simulink model "ResonantConverter_GaN"  (R2016a)
settings: Solver=VariableStepAuto  StartTime=0.0  StopTime=0.1  FixedStep=1e-6  RelTol=1e-3
libraries: powerlib x142, dspstat3 x22, powerlib_meascontrol x13
(part 1 of 2)
settings Model: Creator=syf  LastModifiedBy=syf
settings SolverCC: AutoInsertRateTranBlk=on

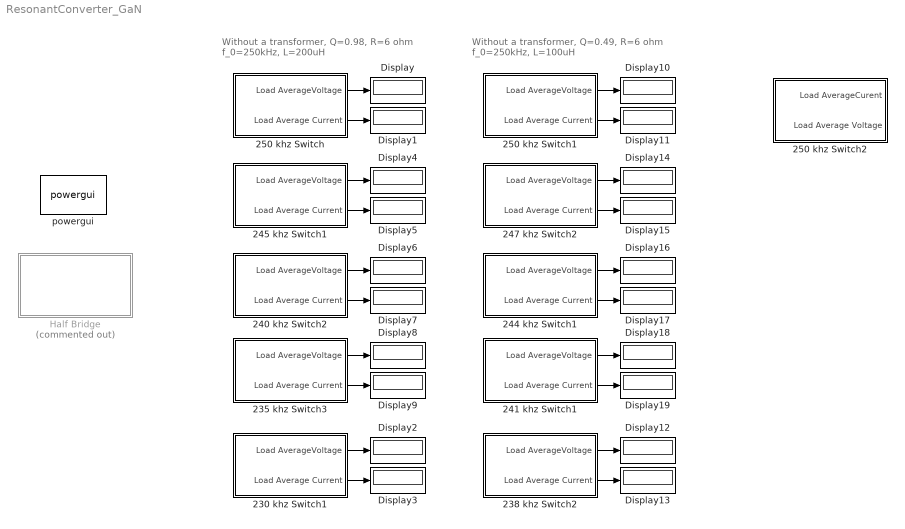
== system ResonantConverter_GaN ==
  note: Without a transformer, Q=0.98, R=6 ohm
      | f_0=250kHz, L=200uH
  note: Without a transformer, Q=0.49, R=6 ohm
      | f_0=250kHz, L=100uH
  230 khz Switch1 : Subsystem
  235 khz Switch3 : Subsystem
  238 khz Switch2 : Subsystem
  240 khz Switch2 : Subsystem
  241 khz Switch1 : Subsystem
  244 khz Switch1 : Subsystem
  245 khz Switch1 : Subsystem
  247 khz Switch2 : Subsystem
  250 khz Switch : Subsystem
  250 khz Switch1 : Subsystem
  250 khz Switch2 : Subsystem
  Display{,1..19} (20 alike) : Display
  Half Bridge : Subsystem  Commented=on
  powergui : powerlib/powergui  Priority=1  SimulationMode=Continuous  SolverType=Tustin/Backward Euler (TBE)  SampleTime=50e-6  frequency=60  SPID=on  DisableSnubberDevices=on  DisableRonSwitches=off  DisableVfSwitches=off  SwTol=0  DisplayEquations=off  Interpol=off  ExternalGateDelay=off  methode=off  Ts=10  FunctionMessages=off  echomessages=off  HookPort=off  EnableUseOfTLC=off  x0status=blocks  frequencyindice=0  Pbase=100e6  ErrMax=1e-4  Iterations=50  UnitsV=kV  UnitsW=MW  buscounter=0  RestoreLinks=warning  ResistiveCurrentMeasurement=off  Frange=[0:2:500]  Ylog=off  Xlog=on  ShowGrid=off  save=off  variable=ZData  structure=0  ZoomFFT=off  StartTime=0.0  cycles=1  DisplayStyle=1  fundamental=60  FreqAxis=off  MaxFrequency=1000  frequencyindicesteady=1  RmsSteady=1  display=off
  wires:
  250 khz Switch/2(Load Average Current) -> Display1/1
  250 khz Switch/1(Load AverageVoltage) -> Display/1
  230 khz Switch1/2(Load Average Current) -> Display3/1
  230 khz Switch1/1(Load AverageVoltage) -> Display2/1
  245 khz Switch1/2(Load Average Current) -> Display5/1
  245 khz Switch1/1(Load AverageVoltage) -> Display4/1
  240 khz Switch2/2(Load Average Current) -> Display7/1
  240 khz Switch2/1(Load AverageVoltage) -> Display6/1
  235 khz Switch3/2(Load Average Current) -> Display9/1
  235 khz Switch3/1(Load AverageVoltage) -> Display8/1
  250 khz Switch1/2(Load Average Current) -> Display11/1
  250 khz Switch1/1(Load AverageVoltage) -> Display10/1
  238 khz Switch2/2(Load Average Current) -> Display13/1
  238 khz Switch2/1(Load AverageVoltage) -> Display12/1
  247 khz Switch2/2(Load Average Current) -> Display15/1
  247 khz Switch2/1(Load AverageVoltage) -> Display14/1
  244 khz Switch1/2(Load Average Current) -> Display17/1
  244 khz Switch1/1(Load AverageVoltage) -> Display16/1
  241 khz Switch1/2(Load Average Current) -> Display19/1
  241 khz Switch1/1(Load AverageVoltage) -> Display18/1

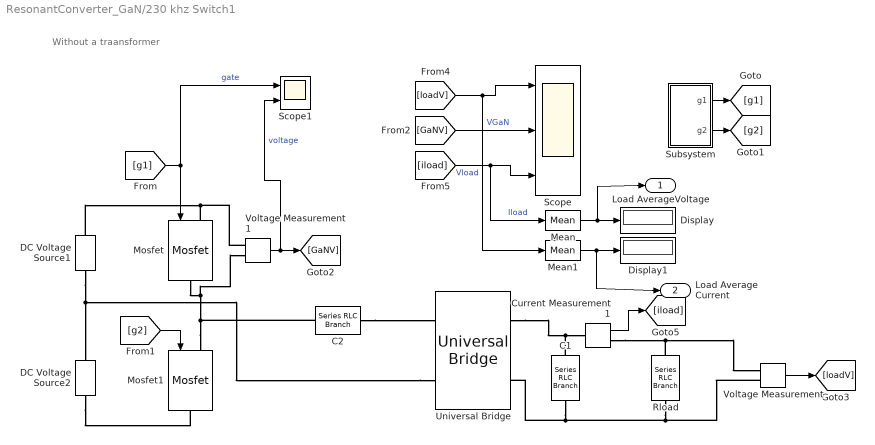
== system ResonantConverter_GaN/230 khz Switch1 ==
  note: Without a traansformer
  C1 : powerlib/Elements/Series RLC Branch  LConnTagsString=__new0  RConnTagsString=__new0  BranchType=C  Resistance=1  Inductance=1e-3  SetiL0=off  InitialCurrent=0  Capacitance=47e-6  Setx0=off  InitialVoltage=0  Measurements=None
  C2 : powerlib/Elements/Series RLC Branch  LConnTagsString=__new0  RConnTagsString=__new0  BranchType=LC  Resistance=1  Inductance=200e-6  SetiL0=off  InitialCurrent=0  Capacitance=0.02027e-7  Setx0=off  InitialVoltage=0  Measurements=None
  Current Measurement1 : powerlib/Measurements/Current Measurement  PhasorSimulation=off  OutputType=Complex  PSBequivalent=0
  DC Voltage Source1 : powerlib/Electrical Sources/DC Voltage Source  Amplitude=190  Measurements=None
  DC Voltage Source2 : powerlib/Electrical Sources/DC Voltage Source  Amplitude=190  Measurements=None
  Display : Display
  Display1 : Display
  Mean : dspstat3/Mean  run=off  reset_popup=None  InputProcessing=Columns as channels (frame based)  directionMode=Each column  dimension=1  roiEnable=off  roiType=Rectangles  roiPortion=Entire ROI  roiOutput=Individual statistics for each ROI  roiFlag=off  outputDataTypeStr=Inherit: Same as accumulator  outputLastDataTypeStr=Inherit: Same as accumulator  outputMin=[]  outputMax=[]  roundingMode=Floor  overflowMode=off
  Mean1 : dspstat3/Mean  run=off  reset_popup=None  InputProcessing=Columns as channels (frame based)  directionMode=Each column  dimension=1  roiEnable=off  roiType=Rectangles  roiPortion=Entire ROI  roiOutput=Individual statistics for each ROI  roiFlag=off  outputDataTypeStr=Inherit: Same as accumulator  outputLastDataTypeStr=Inherit: Same as accumulator  outputMin=[]  outputMax=[]  roundingMode=Floor  overflowMode=off
  Mosfet : powerlib/Power Electronics/Mosfet  Ron=130e-3  Lon=0  Rd=0.25  Vfd=2.2  IC=0  Rs=1e5  Cs=inf  Measurements=off
  Mosfet1 : powerlib/Power Electronics/Mosfet  Ron=130e-3  Lon=0  Rd=0.25  Vfd=2.2  IC=0  Rs=1e5  Cs=inf  Measurements=off
  Rload : powerlib/Elements/Series RLC Branch  LConnTagsString=__new0  RConnTagsString=__new0  BranchType=R  Resistance=6  Inductance=1e-3  SetiL0=off  InitialCurrent=0  Capacitance=1e-6  Setx0=off  InitialVoltage=0  Measurements=None
  Scope : Scope  NumInputPorts=3
  Scope1 : Scope  NumInputPorts=2
  Subsystem : Subsystem
  Universal Bridge : powerlib/Power Electronics/Universal Bridge  Arms=2  SnubberResistance=1e5  SnubberCapacitance=inf  Device=Diodes  Ron=1e-3  Lon=0  ForwardVoltages="[  0  0  ]"  ForwardVoltage=0  GTOparameters=[ 10e-6 , 20e-6 ]  IGBTparameters=[ 1e-6 , 2e-6 ]  Measurements=None  Measurements_2=None  converterType=Rectifier
  Voltage Measurement : powerlib/Measurements/Voltage Measurement  PhasorSimulation=off  OutputType=Complex  PSBequivalent=0
  Voltage Measurement1 : powerlib/Measurements/Voltage Measurement  PhasorSimulation=off  OutputType=Complex  PSBequivalent=0
  Load AverageVoltage : Outport
  Load Average Current : Outport  Port=2
  wires:
  Mean1/1 -> Display1/1, Load Average Current/1
  Current Measurement1/1 -> [iload]
  Voltage Measurement1/1 -> Scope1/2, [GaNV]  "voltage"
  [g2] -> Mosfet1/1
  Voltage Measurement/1 -> [loadV]
  [GaNV] -> Scope/2  "VGaN"
  [loadV] -> Scope/1, Mean1/1  "Vload"
  [iload] -> Scope/3, Mean/1  "Iload"
  [g1] -> Scope1/1, Mosfet/1  "gate"
  Subsystem/2(g2) -> [g2]
  Subsystem/1("g1 ") -> [g1]
  Mean/1 -> Display/1, Load AverageVoltage/1
  connections:
  DC Voltage Source2/LConn1 -- Mosfet1/RConn1
  Current Measurement1/RConn1 -- Voltage Measurement/LConn1 -- Rload/LConn1
  Universal Bridge/LConn2 -- DC Voltage Source1/LConn1 -- DC Voltage Source2/RConn1
  DC Voltage Source1/RConn1 -- Voltage Measurement1/LConn1 -- Mosfet/LConn1
  Mosfet1/LConn1 -- C2/LConn1 -- Voltage Measurement1/LConn2 -- Mosfet/RConn1
  C1/LConn1 -- Universal Bridge/RConn1 -- Current Measurement1/LConn1
  C1/RConn1 -- Universal Bridge/RConn2 -- Voltage Measurement/LConn2 -- Rload/RConn1
  C2/RConn1 -- Universal Bridge/LConn1

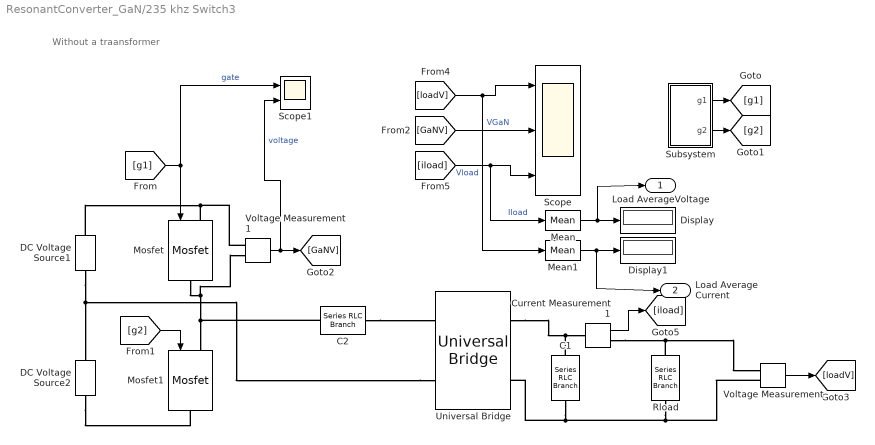
== system ResonantConverter_GaN/235 khz Switch3 ==
  note: Without a traansformer
  C1 : powerlib/Elements/Series RLC Branch  LConnTagsString=__new0  RConnTagsString=__new0  BranchType=C  Resistance=1  Inductance=1e-3  SetiL0=off  InitialCurrent=0  Capacitance=47e-6  Setx0=off  InitialVoltage=0  Measurements=None
  C2 : powerlib/Elements/Series RLC Branch  LConnTagsString=__new0  RConnTagsString=__new0  BranchType=LC  Resistance=1  Inductance=200e-6  SetiL0=off  InitialCurrent=0  Capacitance=0.02027e-7  Setx0=off  InitialVoltage=0  Measurements=None
  Current Measurement1 : powerlib/Measurements/Current Measurement  PhasorSimulation=off  OutputType=Complex  PSBequivalent=0
  DC Voltage Source1 : powerlib/Electrical Sources/DC Voltage Source  Amplitude=190  Measurements=None
  DC Voltage Source2 : powerlib/Electrical Sources/DC Voltage Source  Amplitude=190  Measurements=None
  Display : Display
  Display1 : Display
  Mean : dspstat3/Mean  run=off  reset_popup=None  InputProcessing=Columns as channels (frame based)  directionMode=Each column  dimension=1  roiEnable=off  roiType=Rectangles  roiPortion=Entire ROI  roiOutput=Individual statistics for each ROI  roiFlag=off  outputDataTypeStr=Inherit: Same as accumulator  outputLastDataTypeStr=Inherit: Same as accumulator  outputMin=[]  outputMax=[]  roundingMode=Floor  overflowMode=off
  Mean1 : dspstat3/Mean  run=off  reset_popup=None  InputProcessing=Columns as channels (frame based)  directionMode=Each column  dimension=1  roiEnable=off  roiType=Rectangles  roiPortion=Entire ROI  roiOutput=Individual statistics for each ROI  roiFlag=off  outputDataTypeStr=Inherit: Same as accumulator  outputLastDataTypeStr=Inherit: Same as accumulator  outputMin=[]  outputMax=[]  roundingMode=Floor  overflowMode=off
  Mosfet : powerlib/Power Electronics/Mosfet  Ron=130e-3  Lon=0  Rd=0.25  Vfd=2.2  IC=0  Rs=1e5  Cs=inf  Measurements=off
  Mosfet1 : powerlib/Power Electronics/Mosfet  Ron=130e-3  Lon=0  Rd=0.25  Vfd=2.2  IC=0  Rs=1e5  Cs=inf  Measurements=off
  Rload : powerlib/Elements/Series RLC Branch  LConnTagsString=__new0  RConnTagsString=__new0  BranchType=R  Resistance=6  Inductance=1e-3  SetiL0=off  InitialCurrent=0  Capacitance=1e-6  Setx0=off  InitialVoltage=0  Measurements=None
  Scope : Scope  NumInputPorts=3
  Scope1 : Scope  NumInputPorts=2
  Subsystem : Subsystem
  Universal Bridge : powerlib/Power Electronics/Universal Bridge  Arms=2  SnubberResistance=1e5  SnubberCapacitance=inf  Device=Diodes  Ron=1e-3  Lon=0  ForwardVoltages="[  0  0  ]"  ForwardVoltage=0  GTOparameters=[ 10e-6 , 20e-6 ]  IGBTparameters=[ 1e-6 , 2e-6 ]  Measurements=None  Measurements_2=None  converterType=Rectifier
  Voltage Measurement : powerlib/Measurements/Voltage Measurement  PhasorSimulation=off  OutputType=Complex  PSBequivalent=0
  Voltage Measurement1 : powerlib/Measurements/Voltage Measurement  PhasorSimulation=off  OutputType=Complex  PSBequivalent=0
  Load AverageVoltage : Outport
  Load Average Current : Outport  Port=2
  wires:
  Mean1/1 -> Display1/1, Load Average Current/1
  Current Measurement1/1 -> [iload]
  Voltage Measurement1/1 -> Scope1/2, [GaNV]  "voltage"
  [g2] -> Mosfet1/1
  Voltage Measurement/1 -> [loadV]
  [GaNV] -> Scope/2  "VGaN"
  [loadV] -> Scope/1, Mean1/1  "Vload"
  [iload] -> Scope/3, Mean/1  "Iload"
  [g1] -> Scope1/1, Mosfet/1  "gate"
  Subsystem/2(g2) -> [g2]
  Subsystem/1("g1 ") -> [g1]
  Mean/1 -> Display/1, Load AverageVoltage/1
  connections:
  DC Voltage Source2/LConn1 -- Mosfet1/RConn1
  Current Measurement1/RConn1 -- Voltage Measurement/LConn1 -- Rload/LConn1
  Universal Bridge/LConn2 -- DC Voltage Source1/LConn1 -- DC Voltage Source2/RConn1
  DC Voltage Source1/RConn1 -- Voltage Measurement1/LConn1 -- Mosfet/LConn1
  C2/LConn1 -- Mosfet1/LConn1 -- Voltage Measurement1/LConn2 -- Mosfet/RConn1
  C1/LConn1 -- Universal Bridge/RConn1 -- Current Measurement1/LConn1
  C1/RConn1 -- Universal Bridge/RConn2 -- Voltage Measurement/LConn2 -- Rload/RConn1
  C2/RConn1 -- Universal Bridge/LConn1

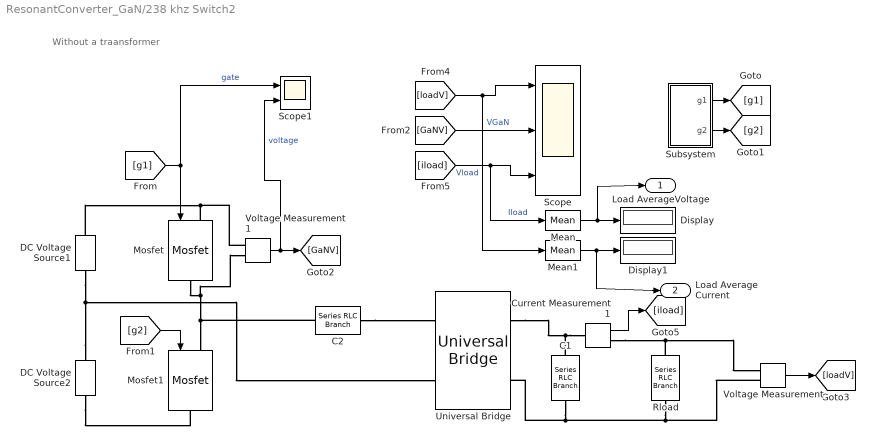
== system ResonantConverter_GaN/238 khz Switch2 ==
  note: Without a traansformer
  C1 : powerlib/Elements/Series RLC Branch  LConnTagsString=__new0  RConnTagsString=__new0  BranchType=C  Resistance=1  Inductance=1e-3  SetiL0=off  InitialCurrent=0  Capacitance=47e-6  Setx0=off  InitialVoltage=0  Measurements=None
  C2 : powerlib/Elements/Series RLC Branch  LConnTagsString=__new0  RConnTagsString=__new0  BranchType=LC  Resistance=1  Inductance=100e-6  SetiL0=off  InitialCurrent=0  Capacitance=0.02027e-7*2  Setx0=off  InitialVoltage=0  Measurements=None
  Current Measurement1 : powerlib/Measurements/Current Measurement  PhasorSimulation=off  OutputType=Complex  PSBequivalent=0
  DC Voltage Source1 : powerlib/Electrical Sources/DC Voltage Source  Amplitude=190  Measurements=None
  DC Voltage Source2 : powerlib/Electrical Sources/DC Voltage Source  Amplitude=190  Measurements=None
  Display : Display
  Display1 : Display
  Mean : dspstat3/Mean  run=off  reset_popup=None  InputProcessing=Columns as channels (frame based)  directionMode=Each column  dimension=1  roiEnable=off  roiType=Rectangles  roiPortion=Entire ROI  roiOutput=Individual statistics for each ROI  roiFlag=off  outputDataTypeStr=Inherit: Same as accumulator  outputLastDataTypeStr=Inherit: Same as accumulator  outputMin=[]  outputMax=[]  roundingMode=Floor  overflowMode=off
  Mean1 : dspstat3/Mean  run=off  reset_popup=None  InputProcessing=Columns as channels (frame based)  directionMode=Each column  dimension=1  roiEnable=off  roiType=Rectangles  roiPortion=Entire ROI  roiOutput=Individual statistics for each ROI  roiFlag=off  outputDataTypeStr=Inherit: Same as accumulator  outputLastDataTypeStr=Inherit: Same as accumulator  outputMin=[]  outputMax=[]  roundingMode=Floor  overflowMode=off
  Mosfet : powerlib/Power Electronics/Mosfet  Ron=130e-3  Lon=0  Rd=0.25  Vfd=2.2  IC=0  Rs=1e5  Cs=inf  Measurements=off
  Mosfet1 : powerlib/Power Electronics/Mosfet  Ron=130e-3  Lon=0  Rd=0.25  Vfd=2.2  IC=0  Rs=1e5  Cs=inf  Measurements=off
  Rload : powerlib/Elements/Series RLC Branch  LConnTagsString=__new0  RConnTagsString=__new0  BranchType=R  Resistance=6  Inductance=1e-3  SetiL0=off  InitialCurrent=0  Capacitance=1e-6  Setx0=off  InitialVoltage=0  Measurements=None
  Scope : Scope  NumInputPorts=3
  Scope1 : Scope  NumInputPorts=2
  Subsystem : Subsystem
  Universal Bridge : powerlib/Power Electronics/Universal Bridge  Arms=2  SnubberResistance=1e5  SnubberCapacitance=inf  Device=Diodes  Ron=1e-3  Lon=0  ForwardVoltages="[  0  0  ]"  ForwardVoltage=0  GTOparameters=[ 10e-6 , 20e-6 ]  IGBTparameters=[ 1e-6 , 2e-6 ]  Measurements=None  Measurements_2=None  converterType=Rectifier
  Voltage Measurement : powerlib/Measurements/Voltage Measurement  PhasorSimulation=off  OutputType=Complex  PSBequivalent=0
  Voltage Measurement1 : powerlib/Measurements/Voltage Measurement  PhasorSimulation=off  OutputType=Complex  PSBequivalent=0
  Load AverageVoltage : Outport
  Load Average Current : Outport  Port=2
  wires:
  Mean/1 -> Load AverageVoltage/1, Display/1
  Subsystem/1("g1 ") -> [g1]
  Subsystem/2(g2) -> [g2]
  [g1] -> Mosfet/1, Scope1/1  "gate"
  [iload] -> Mean/1, Scope/3  "Iload"
  [loadV] -> Mean1/1, Scope/1  "Vload"
  [GaNV] -> Scope/2  "VGaN"
  Voltage Measurement/1 -> [loadV]
  [g2] -> Mosfet1/1
  Voltage Measurement1/1 -> [GaNV], Scope1/2  "voltage"
  Current Measurement1/1 -> [iload]
  Mean1/1 -> Load Average Current/1, Display1/1
  connections:
  C2/RConn1 -- Universal Bridge/LConn1
  Rload/RConn1 -- Voltage Measurement/LConn2 -- Universal Bridge/RConn2 -- C1/RConn1
  Current Measurement1/LConn1 -- Universal Bridge/RConn1 -- C1/LConn1
  Mosfet/RConn1 -- Voltage Measurement1/LConn2 -- C2/LConn1 -- Mosfet1/LConn1
  Mosfet/LConn1 -- Voltage Measurement1/LConn1 -- DC Voltage Source1/RConn1
  DC Voltage Source2/RConn1 -- DC Voltage Source1/LConn1 -- Universal Bridge/LConn2
  Rload/LConn1 -- Voltage Measurement/LConn1 -- Current Measurement1/RConn1
  DC Voltage Source2/LConn1 -- Mosfet1/RConn1

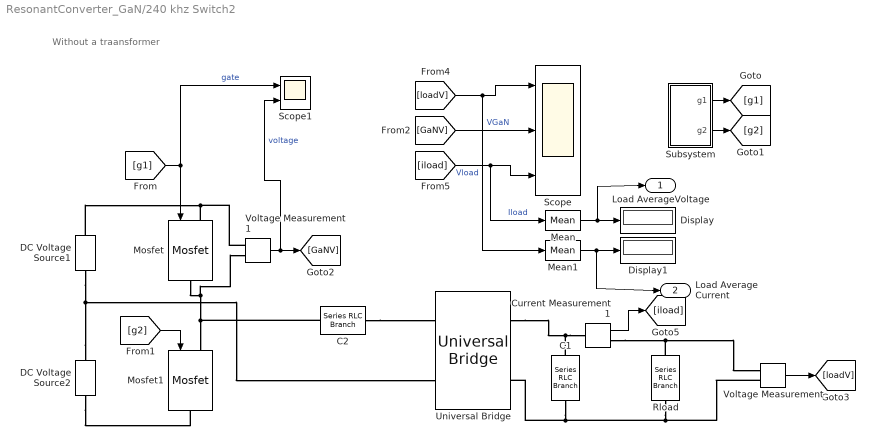
== system ResonantConverter_GaN/240 khz Switch2 ==
  note: Without a traansformer
  C1 : powerlib/Elements/Series RLC Branch  LConnTagsString=__new0  RConnTagsString=__new0  BranchType=C  Resistance=1  Inductance=1e-3  SetiL0=off  InitialCurrent=0  Capacitance=47e-6  Setx0=off  InitialVoltage=0  Measurements=None
  C2 : powerlib/Elements/Series RLC Branch  LConnTagsString=__new0  RConnTagsString=__new0  BranchType=LC  Resistance=1  Inductance=200e-6  SetiL0=off  InitialCurrent=0  Capacitance=0.02027e-7  Setx0=off  InitialVoltage=0  Measurements=None
  Current Measurement1 : powerlib/Measurements/Current Measurement  PhasorSimulation=off  OutputType=Complex  PSBequivalent=0
  DC Voltage Source1 : powerlib/Electrical Sources/DC Voltage Source  Amplitude=190  Measurements=None
  DC Voltage Source2 : powerlib/Electrical Sources/DC Voltage Source  Amplitude=190  Measurements=None
  Display : Display
  Display1 : Display
  Mean : dspstat3/Mean  run=off  reset_popup=None  InputProcessing=Columns as channels (frame based)  directionMode=Each column  dimension=1  roiEnable=off  roiType=Rectangles  roiPortion=Entire ROI  roiOutput=Individual statistics for each ROI  roiFlag=off  outputDataTypeStr=Inherit: Same as accumulator  outputLastDataTypeStr=Inherit: Same as accumulator  outputMin=[]  outputMax=[]  roundingMode=Floor  overflowMode=off
  Mean1 : dspstat3/Mean  run=off  reset_popup=None  InputProcessing=Columns as channels (frame based)  directionMode=Each column  dimension=1  roiEnable=off  roiType=Rectangles  roiPortion=Entire ROI  roiOutput=Individual statistics for each ROI  roiFlag=off  outputDataTypeStr=Inherit: Same as accumulator  outputLastDataTypeStr=Inherit: Same as accumulator  outputMin=[]  outputMax=[]  roundingMode=Floor  overflowMode=off
  Mosfet : powerlib/Power Electronics/Mosfet  Ron=130e-3  Lon=0  Rd=0.25  Vfd=2.2  IC=0  Rs=1e5  Cs=inf  Measurements=off
  Mosfet1 : powerlib/Power Electronics/Mosfet  Ron=130e-3  Lon=0  Rd=0.25  Vfd=2.2  IC=0  Rs=1e5  Cs=inf  Measurements=off
  Rload : powerlib/Elements/Series RLC Branch  LConnTagsString=__new0  RConnTagsString=__new0  BranchType=R  Resistance=6  Inductance=1e-3  SetiL0=off  InitialCurrent=0  Capacitance=1e-6  Setx0=off  InitialVoltage=0  Measurements=None
  Scope : Scope  NumInputPorts=3
  Scope1 : Scope  NumInputPorts=2
  Subsystem : Subsystem
  Universal Bridge : powerlib/Power Electronics/Universal Bridge  Arms=2  SnubberResistance=1e5  SnubberCapacitance=inf  Device=Diodes  Ron=1e-3  Lon=0  ForwardVoltages="[  0  0  ]"  ForwardVoltage=0  GTOparameters=[ 10e-6 , 20e-6 ]  IGBTparameters=[ 1e-6 , 2e-6 ]  Measurements=None  Measurements_2=None  converterType=Rectifier
  Voltage Measurement : powerlib/Measurements/Voltage Measurement  PhasorSimulation=off  OutputType=Complex  PSBequivalent=0
  Voltage Measurement1 : powerlib/Measurements/Voltage Measurement  PhasorSimulation=off  OutputType=Complex  PSBequivalent=0
  Load AverageVoltage : Outport
  Load Average Current : Outport  Port=2
  wires:
  Mean/1 -> Load AverageVoltage/1, Display/1
  Subsystem/1("g1 ") -> [g1]
  Subsystem/2(g2) -> [g2]
  [g1] -> Mosfet/1, Scope1/1  "gate"
  [iload] -> Mean/1, Scope/3  "Iload"
  [loadV] -> Mean1/1, Scope/1  "Vload"
  [GaNV] -> Scope/2  "VGaN"
  Voltage Measurement/1 -> [loadV]
  [g2] -> Mosfet1/1
  Voltage Measurement1/1 -> [GaNV], Scope1/2  "voltage"
  Current Measurement1/1 -> [iload]
  Mean1/1 -> Load Average Current/1, Display1/1
  connections:
  C2/RConn1 -- Universal Bridge/LConn1
  Rload/RConn1 -- Voltage Measurement/LConn2 -- Universal Bridge/RConn2 -- C1/RConn1
  Current Measurement1/LConn1 -- Universal Bridge/RConn1 -- C1/LConn1
  Mosfet/RConn1 -- Voltage Measurement1/LConn2 -- Mosfet1/LConn1 -- C2/LConn1
  Mosfet/LConn1 -- Voltage Measurement1/LConn1 -- DC Voltage Source1/RConn1
  DC Voltage Source2/RConn1 -- DC Voltage Source1/LConn1 -- Universal Bridge/LConn2
  Rload/LConn1 -- Voltage Measurement/LConn1 -- Current Measurement1/RConn1
  DC Voltage Source2/LConn1 -- Mosfet1/RConn1

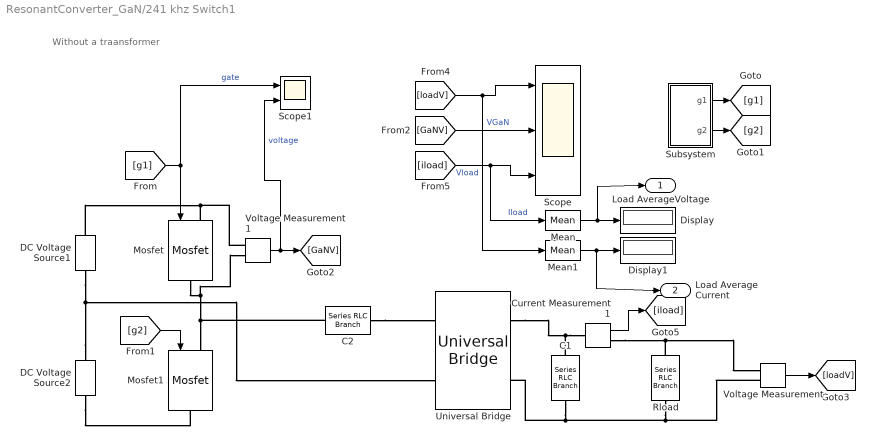
== system ResonantConverter_GaN/241 khz Switch1 ==
  note: Without a traansformer
  C1 : powerlib/Elements/Series RLC Branch  LConnTagsString=__new0  RConnTagsString=__new0  BranchType=C  Resistance=1  Inductance=1e-3  SetiL0=off  InitialCurrent=0  Capacitance=47e-6  Setx0=off  InitialVoltage=0  Measurements=None
  C2 : powerlib/Elements/Series RLC Branch  LConnTagsString=__new0  RConnTagsString=__new0  BranchType=LC  Resistance=1  Inductance=100e-6  SetiL0=off  InitialCurrent=0  Capacitance=0.02027e-7*2  Setx0=off  InitialVoltage=0  Measurements=None
  Current Measurement1 : powerlib/Measurements/Current Measurement  PhasorSimulation=off  OutputType=Complex  PSBequivalent=0
  DC Voltage Source1 : powerlib/Electrical Sources/DC Voltage Source  Amplitude=190  Measurements=None
  DC Voltage Source2 : powerlib/Electrical Sources/DC Voltage Source  Amplitude=190  Measurements=None
  Display : Display
  Display1 : Display
  Mean : dspstat3/Mean  run=off  reset_popup=None  InputProcessing=Columns as channels (frame based)  directionMode=Each column  dimension=1  roiEnable=off  roiType=Rectangles  roiPortion=Entire ROI  roiOutput=Individual statistics for each ROI  roiFlag=off  outputDataTypeStr=Inherit: Same as accumulator  outputLastDataTypeStr=Inherit: Same as accumulator  outputMin=[]  outputMax=[]  roundingMode=Floor  overflowMode=off
  Mean1 : dspstat3/Mean  run=off  reset_popup=None  InputProcessing=Columns as channels (frame based)  directionMode=Each column  dimension=1  roiEnable=off  roiType=Rectangles  roiPortion=Entire ROI  roiOutput=Individual statistics for each ROI  roiFlag=off  outputDataTypeStr=Inherit: Same as accumulator  outputLastDataTypeStr=Inherit: Same as accumulator  outputMin=[]  outputMax=[]  roundingMode=Floor  overflowMode=off
  Mosfet : powerlib/Power Electronics/Mosfet  Ron=130e-3  Lon=0  Rd=0.25  Vfd=2.2  IC=0  Rs=1e5  Cs=inf  Measurements=off
  Mosfet1 : powerlib/Power Electronics/Mosfet  Ron=130e-3  Lon=0  Rd=0.25  Vfd=2.2  IC=0  Rs=1e5  Cs=inf  Measurements=off
  Rload : powerlib/Elements/Series RLC Branch  LConnTagsString=__new0  RConnTagsString=__new0  BranchType=R  Resistance=6  Inductance=1e-3  SetiL0=off  InitialCurrent=0  Capacitance=1e-6  Setx0=off  InitialVoltage=0  Measurements=None
  Scope : Scope  NumInputPorts=3
  Scope1 : Scope  NumInputPorts=2
  Subsystem : Subsystem
  Universal Bridge : powerlib/Power Electronics/Universal Bridge  Arms=2  SnubberResistance=1e5  SnubberCapacitance=inf  Device=Diodes  Ron=1e-3  Lon=0  ForwardVoltages="[  0  0  ]"  ForwardVoltage=0  GTOparameters=[ 10e-6 , 20e-6 ]  IGBTparameters=[ 1e-6 , 2e-6 ]  Measurements=None  Measurements_2=None  converterType=Rectifier
  Voltage Measurement : powerlib/Measurements/Voltage Measurement  PhasorSimulation=off  OutputType=Complex  PSBequivalent=0
  Voltage Measurement1 : powerlib/Measurements/Voltage Measurement  PhasorSimulation=off  OutputType=Complex  PSBequivalent=0
  Load AverageVoltage : Outport
  Load Average Current : Outport  Port=2
  wires:
  Mean/1 -> Load AverageVoltage/1, Display/1
  Subsystem/1("g1 ") -> [g1]
  Subsystem/2(g2) -> [g2]
  [g1] -> Mosfet/1, Scope1/1  "gate"
  [iload] -> Mean/1, Scope/3  "Iload"
  [loadV] -> Mean1/1, Scope/1  "Vload"
  [GaNV] -> Scope/2  "VGaN"
  Voltage Measurement/1 -> [loadV]
  [g2] -> Mosfet1/1
  Voltage Measurement1/1 -> [GaNV], Scope1/2  "voltage"
  Current Measurement1/1 -> [iload]
  Mean1/1 -> Load Average Current/1, Display1/1
  connections:
  C2/RConn1 -- Universal Bridge/LConn1
  Rload/RConn1 -- Voltage Measurement/LConn2 -- Universal Bridge/RConn2 -- C1/RConn1
  Current Measurement1/LConn1 -- Universal Bridge/RConn1 -- C1/LConn1
  Mosfet/RConn1 -- Voltage Measurement1/LConn2 -- C2/LConn1 -- Mosfet1/LConn1
  Mosfet/LConn1 -- Voltage Measurement1/LConn1 -- DC Voltage Source1/RConn1
  DC Voltage Source2/RConn1 -- DC Voltage Source1/LConn1 -- Universal Bridge/LConn2
  Rload/LConn1 -- Voltage Measurement/LConn1 -- Current Measurement1/RConn1
  DC Voltage Source2/LConn1 -- Mosfet1/RConn1

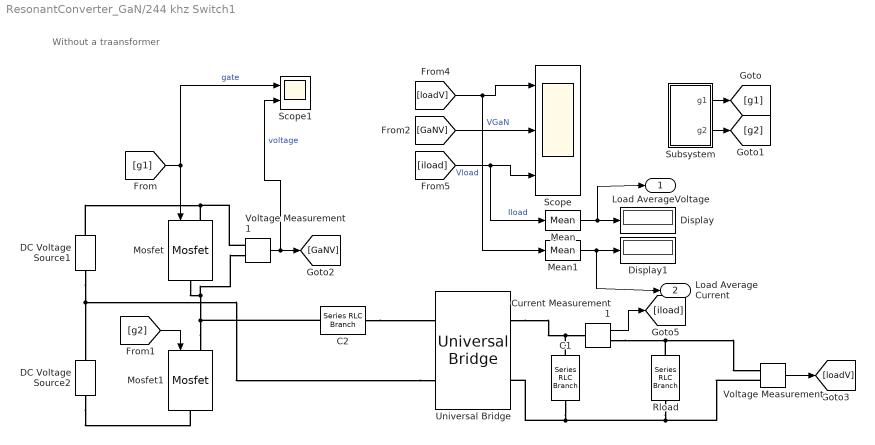
== system ResonantConverter_GaN/244 khz Switch1 ==
  note: Without a traansformer
  C1 : powerlib/Elements/Series RLC Branch  LConnTagsString=__new0  RConnTagsString=__new0  BranchType=C  Resistance=1  Inductance=1e-3  SetiL0=off  InitialCurrent=0  Capacitance=47e-6  Setx0=off  InitialVoltage=0  Measurements=None
  C2 : powerlib/Elements/Series RLC Branch  LConnTagsString=__new0  RConnTagsString=__new0  BranchType=LC  Resistance=1  Inductance=100e-6  SetiL0=off  InitialCurrent=0  Capacitance=0.02027e-7*2  Setx0=off  InitialVoltage=0  Measurements=None
  Current Measurement1 : powerlib/Measurements/Current Measurement  PhasorSimulation=off  OutputType=Complex  PSBequivalent=0
  DC Voltage Source1 : powerlib/Electrical Sources/DC Voltage Source  Amplitude=190  Measurements=None
  DC Voltage Source2 : powerlib/Electrical Sources/DC Voltage Source  Amplitude=190  Measurements=None
  Display : Display
  Display1 : Display
  Mean : dspstat3/Mean  run=off  reset_popup=None  InputProcessing=Columns as channels (frame based)  directionMode=Each column  dimension=1  roiEnable=off  roiType=Rectangles  roiPortion=Entire ROI  roiOutput=Individual statistics for each ROI  roiFlag=off  outputDataTypeStr=Inherit: Same as accumulator  outputLastDataTypeStr=Inherit: Same as accumulator  outputMin=[]  outputMax=[]  roundingMode=Floor  overflowMode=off
  Mean1 : dspstat3/Mean  run=off  reset_popup=None  InputProcessing=Columns as channels (frame based)  directionMode=Each column  dimension=1  roiEnable=off  roiType=Rectangles  roiPortion=Entire ROI  roiOutput=Individual statistics for each ROI  roiFlag=off  outputDataTypeStr=Inherit: Same as accumulator  outputLastDataTypeStr=Inherit: Same as accumulator  outputMin=[]  outputMax=[]  roundingMode=Floor  overflowMode=off
  Mosfet : powerlib/Power Electronics/Mosfet  Ron=130e-3  Lon=0  Rd=0.25  Vfd=2.2  IC=0  Rs=1e5  Cs=inf  Measurements=off
  Mosfet1 : powerlib/Power Electronics/Mosfet  Ron=130e-3  Lon=0  Rd=0.25  Vfd=2.2  IC=0  Rs=1e5  Cs=inf  Measurements=off
  Rload : powerlib/Elements/Series RLC Branch  LConnTagsString=__new0  RConnTagsString=__new0  BranchType=R  Resistance=6  Inductance=1e-3  SetiL0=off  InitialCurrent=0  Capacitance=1e-6  Setx0=off  InitialVoltage=0  Measurements=None
  Scope : Scope  NumInputPorts=3
  Scope1 : Scope  NumInputPorts=2
  Subsystem : Subsystem
  Universal Bridge : powerlib/Power Electronics/Universal Bridge  Arms=2  SnubberResistance=1e5  SnubberCapacitance=inf  Device=Diodes  Ron=1e-3  Lon=0  ForwardVoltages="[  0  0  ]"  ForwardVoltage=0  GTOparameters=[ 10e-6 , 20e-6 ]  IGBTparameters=[ 1e-6 , 2e-6 ]  Measurements=None  Measurements_2=None  converterType=Rectifier
  Voltage Measurement : powerlib/Measurements/Voltage Measurement  PhasorSimulation=off  OutputType=Complex  PSBequivalent=0
  Voltage Measurement1 : powerlib/Measurements/Voltage Measurement  PhasorSimulation=off  OutputType=Complex  PSBequivalent=0
  Load AverageVoltage : Outport
  Load Average Current : Outport  Port=2
  wires:
  Mean1/1 -> Display1/1, Load Average Current/1
  Current Measurement1/1 -> [iload]
  Voltage Measurement1/1 -> Scope1/2, [GaNV]  "voltage"
  [g2] -> Mosfet1/1
  Voltage Measurement/1 -> [loadV]
  [GaNV] -> Scope/2  "VGaN"
  [loadV] -> Scope/1, Mean1/1  "Vload"
  [iload] -> Scope/3, Mean/1  "Iload"
  [g1] -> Scope1/1, Mosfet/1  "gate"
  Subsystem/2(g2) -> [g2]
  Subsystem/1("g1 ") -> [g1]
  Mean/1 -> Display/1, Load AverageVoltage/1
  connections:
  DC Voltage Source2/LConn1 -- Mosfet1/RConn1
  Current Measurement1/RConn1 -- Voltage Measurement/LConn1 -- Rload/LConn1
  Universal Bridge/LConn2 -- DC Voltage Source1/LConn1 -- DC Voltage Source2/RConn1
  DC Voltage Source1/RConn1 -- Voltage Measurement1/LConn1 -- Mosfet/LConn1
  Mosfet1/LConn1 -- C2/LConn1 -- Voltage Measurement1/LConn2 -- Mosfet/RConn1
  C1/LConn1 -- Universal Bridge/RConn1 -- Current Measurement1/LConn1
  C1/RConn1 -- Universal Bridge/RConn2 -- Voltage Measurement/LConn2 -- Rload/RConn1
  C2/RConn1 -- Universal Bridge/LConn1

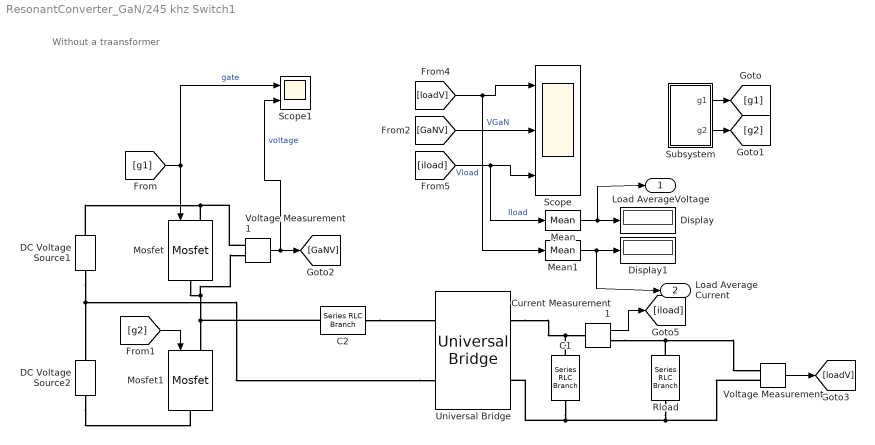
== system ResonantConverter_GaN/245 khz Switch1 ==
  note: Without a traansformer
  C1 : powerlib/Elements/Series RLC Branch  LConnTagsString=__new0  RConnTagsString=__new0  BranchType=C  Resistance=1  Inductance=1e-3  SetiL0=off  InitialCurrent=0  Capacitance=47e-6  Setx0=off  InitialVoltage=0  Measurements=None
  C2 : powerlib/Elements/Series RLC Branch  LConnTagsString=__new0  RConnTagsString=__new0  BranchType=LC  Resistance=1  Inductance=200e-6  SetiL0=off  InitialCurrent=0  Capacitance=0.02027e-7  Setx0=off  InitialVoltage=0  Measurements=None
  Current Measurement1 : powerlib/Measurements/Current Measurement  PhasorSimulation=off  OutputType=Complex  PSBequivalent=0
  DC Voltage Source1 : powerlib/Electrical Sources/DC Voltage Source  Amplitude=190  Measurements=None
  DC Voltage Source2 : powerlib/Electrical Sources/DC Voltage Source  Amplitude=190  Measurements=None
  Display : Display
  Display1 : Display
  Mean : dspstat3/Mean  run=off  reset_popup=None  InputProcessing=Columns as channels (frame based)  directionMode=Each column  dimension=1  roiEnable=off  roiType=Rectangles  roiPortion=Entire ROI  roiOutput=Individual statistics for each ROI  roiFlag=off  outputDataTypeStr=Inherit: Same as accumulator  outputLastDataTypeStr=Inherit: Same as accumulator  outputMin=[]  outputMax=[]  roundingMode=Floor  overflowMode=off
  Mean1 : dspstat3/Mean  run=off  reset_popup=None  InputProcessing=Columns as channels (frame based)  directionMode=Each column  dimension=1  roiEnable=off  roiType=Rectangles  roiPortion=Entire ROI  roiOutput=Individual statistics for each ROI  roiFlag=off  outputDataTypeStr=Inherit: Same as accumulator  outputLastDataTypeStr=Inherit: Same as accumulator  outputMin=[]  outputMax=[]  roundingMode=Floor  overflowMode=off
  Mosfet : powerlib/Power Electronics/Mosfet  Ron=130e-3  Lon=0  Rd=0.25  Vfd=2.2  IC=0  Rs=1e5  Cs=inf  Measurements=off
  Mosfet1 : powerlib/Power Electronics/Mosfet  Ron=130e-3  Lon=0  Rd=0.25  Vfd=2.2  IC=0  Rs=1e5  Cs=inf  Measurements=off
  Rload : powerlib/Elements/Series RLC Branch  LConnTagsString=__new0  RConnTagsString=__new0  BranchType=R  Resistance=6  Inductance=1e-3  SetiL0=off  InitialCurrent=0  Capacitance=1e-6  Setx0=off  InitialVoltage=0  Measurements=None
  Scope : Scope  NumInputPorts=3
  Scope1 : Scope  NumInputPorts=2
  Subsystem : Subsystem
  Universal Bridge : powerlib/Power Electronics/Universal Bridge  Arms=2  SnubberResistance=1e5  SnubberCapacitance=inf  Device=Diodes  Ron=1e-3  Lon=0  ForwardVoltages="[  0  0  ]"  ForwardVoltage=0  GTOparameters=[ 10e-6 , 20e-6 ]  IGBTparameters=[ 1e-6 , 2e-6 ]  Measurements=None  Measurements_2=None  converterType=Rectifier
  Voltage Measurement : powerlib/Measurements/Voltage Measurement  PhasorSimulation=off  OutputType=Complex  PSBequivalent=0
  Voltage Measurement1 : powerlib/Measurements/Voltage Measurement  PhasorSimulation=off  OutputType=Complex  PSBequivalent=0
  Load AverageVoltage : Outport
  Load Average Current : Outport  Port=2
  wires:
  Mean1/1 -> Display1/1, Load Average Current/1
  Current Measurement1/1 -> [iload]
  Voltage Measurement1/1 -> Scope1/2, [GaNV]  "voltage"
  [g2] -> Mosfet1/1
  Voltage Measurement/1 -> [loadV]
  [GaNV] -> Scope/2  "VGaN"
  [loadV] -> Scope/1, Mean1/1  "Vload"
  [iload] -> Scope/3, Mean/1  "Iload"
  [g1] -> Scope1/1, Mosfet/1  "gate"
  Subsystem/2(g2) -> [g2]
  Subsystem/1("g1 ") -> [g1]
  Mean/1 -> Display/1, Load AverageVoltage/1
  connections:
  DC Voltage Source2/LConn1 -- Mosfet1/RConn1
  Current Measurement1/RConn1 -- Voltage Measurement/LConn1 -- Rload/LConn1
  Universal Bridge/LConn2 -- DC Voltage Source1/LConn1 -- DC Voltage Source2/RConn1
  DC Voltage Source1/RConn1 -- Voltage Measurement1/LConn1 -- Mosfet/LConn1
  C2/LConn1 -- Mosfet1/LConn1 -- Voltage Measurement1/LConn2 -- Mosfet/RConn1
  C1/LConn1 -- Universal Bridge/RConn1 -- Current Measurement1/LConn1
  C1/RConn1 -- Universal Bridge/RConn2 -- Voltage Measurement/LConn2 -- Rload/RConn1
  C2/RConn1 -- Universal Bridge/LConn1

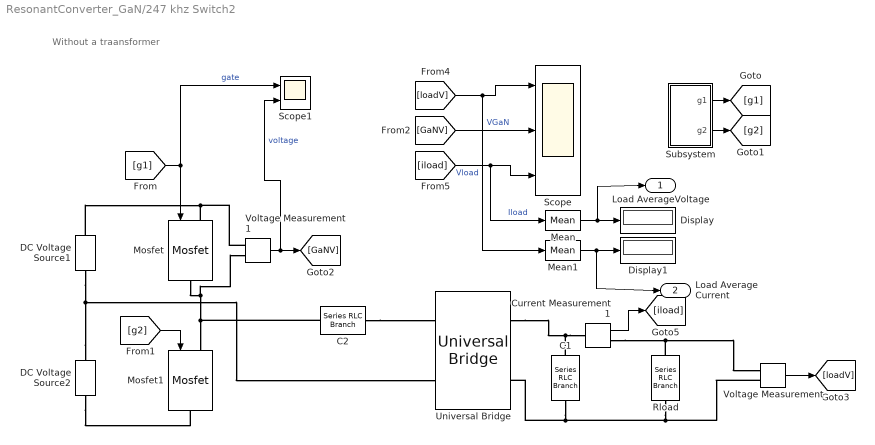
== system ResonantConverter_GaN/247 khz Switch2 ==
  note: Without a traansformer
  C1 : powerlib/Elements/Series RLC Branch  LConnTagsString=__new0  RConnTagsString=__new0  BranchType=C  Resistance=1  Inductance=1e-3  SetiL0=off  InitialCurrent=0  Capacitance=47e-6  Setx0=off  InitialVoltage=0  Measurements=None
  C2 : powerlib/Elements/Series RLC Branch  LConnTagsString=__new0  RConnTagsString=__new0  BranchType=LC  Resistance=1  Inductance=100e-6  SetiL0=off  InitialCurrent=0  Capacitance=0.02027e-7*2  Setx0=off  InitialVoltage=0  Measurements=None
  Current Measurement1 : powerlib/Measurements/Current Measurement  PhasorSimulation=off  OutputType=Complex  PSBequivalent=0
  DC Voltage Source1 : powerlib/Electrical Sources/DC Voltage Source  Amplitude=190  Measurements=None
  DC Voltage Source2 : powerlib/Electrical Sources/DC Voltage Source  Amplitude=190  Measurements=None
  Display : Display
  Display1 : Display
  Mean : dspstat3/Mean  run=off  reset_popup=None  InputProcessing=Columns as channels (frame based)  directionMode=Each column  dimension=1  roiEnable=off  roiType=Rectangles  roiPortion=Entire ROI  roiOutput=Individual statistics for each ROI  roiFlag=off  outputDataTypeStr=Inherit: Same as accumulator  outputLastDataTypeStr=Inherit: Same as accumulator  outputMin=[]  outputMax=[]  roundingMode=Floor  overflowMode=off
  Mean1 : dspstat3/Mean  run=off  reset_popup=None  InputProcessing=Columns as channels (frame based)  directionMode=Each column  dimension=1  roiEnable=off  roiType=Rectangles  roiPortion=Entire ROI  roiOutput=Individual statistics for each ROI  roiFlag=off  outputDataTypeStr=Inherit: Same as accumulator  outputLastDataTypeStr=Inherit: Same as accumulator  outputMin=[]  outputMax=[]  roundingMode=Floor  overflowMode=off
  Mosfet : powerlib/Power Electronics/Mosfet  Ron=130e-3  Lon=0  Rd=0.25  Vfd=2.2  IC=0  Rs=1e5  Cs=inf  Measurements=off
  Mosfet1 : powerlib/Power Electronics/Mosfet  Ron=130e-3  Lon=0  Rd=0.25  Vfd=2.2  IC=0  Rs=1e5  Cs=inf  Measurements=off
  Rload : powerlib/Elements/Series RLC Branch  LConnTagsString=__new0  RConnTagsString=__new0  BranchType=R  Resistance=6  Inductance=1e-3  SetiL0=off  InitialCurrent=0  Capacitance=1e-6  Setx0=off  InitialVoltage=0  Measurements=None
  Scope : Scope  NumInputPorts=3
  Scope1 : Scope  NumInputPorts=2
  Subsystem : Subsystem
  Universal Bridge : powerlib/Power Electronics/Universal Bridge  Arms=2  SnubberResistance=1e5  SnubberCapacitance=inf  Device=Diodes  Ron=1e-3  Lon=0  ForwardVoltages="[  0  0  ]"  ForwardVoltage=0  GTOparameters=[ 10e-6 , 20e-6 ]  IGBTparameters=[ 1e-6 , 2e-6 ]  Measurements=None  Measurements_2=None  converterType=Rectifier
  Voltage Measurement : powerlib/Measurements/Voltage Measurement  PhasorSimulation=off  OutputType=Complex  PSBequivalent=0
  Voltage Measurement1 : powerlib/Measurements/Voltage Measurement  PhasorSimulation=off  OutputType=Complex  PSBequivalent=0
  Load AverageVoltage : Outport
  Load Average Current : Outport  Port=2
  wires:
  Mean/1 -> Load AverageVoltage/1, Display/1
  Subsystem/1("g1 ") -> [g1]
  Subsystem/2(g2) -> [g2]
  [g1] -> Mosfet/1, Scope1/1  "gate"
  [iload] -> Mean/1, Scope/3  "Iload"
  [loadV] -> Mean1/1, Scope/1  "Vload"
  [GaNV] -> Scope/2  "VGaN"
  Voltage Measurement/1 -> [loadV]
  [g2] -> Mosfet1/1
  Voltage Measurement1/1 -> [GaNV], Scope1/2  "voltage"
  Current Measurement1/1 -> [iload]
  Mean1/1 -> Load Average Current/1, Display1/1
  connections:
  C2/RConn1 -- Universal Bridge/LConn1
  Rload/RConn1 -- Voltage Measurement/LConn2 -- Universal Bridge/RConn2 -- C1/RConn1
  Current Measurement1/LConn1 -- Universal Bridge/RConn1 -- C1/LConn1
  Mosfet/RConn1 -- Voltage Measurement1/LConn2 -- C2/LConn1 -- Mosfet1/LConn1
  Mosfet/LConn1 -- Voltage Measurement1/LConn1 -- DC Voltage Source1/RConn1
  DC Voltage Source2/RConn1 -- DC Voltage Source1/LConn1 -- Universal Bridge/LConn2
  Rload/LConn1 -- Voltage Measurement/LConn1 -- Current Measurement1/RConn1
  DC Voltage Source2/LConn1 -- Mosfet1/RConn1

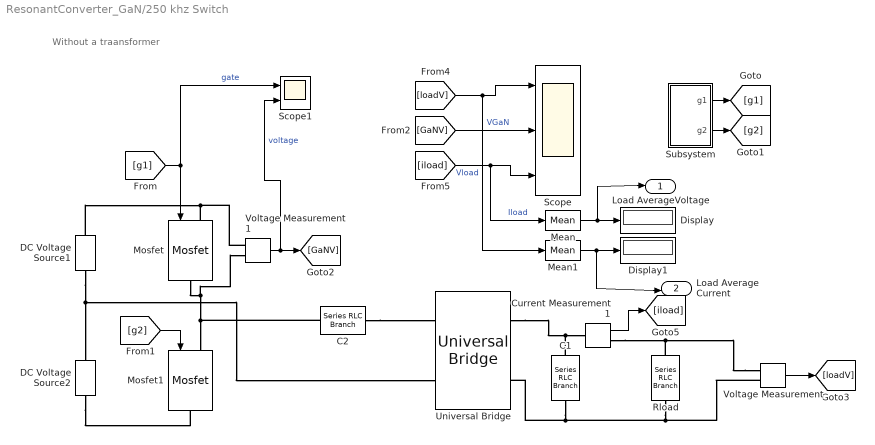
== system ResonantConverter_GaN/250 khz Switch ==
  note: Without a traansformer
  C1 : powerlib/Elements/Series RLC Branch  LConnTagsString=__new0  RConnTagsString=__new0  BranchType=C  Resistance=1  Inductance=1e-3  SetiL0=off  InitialCurrent=0  Capacitance=47e-6  Setx0=off  InitialVoltage=0  Measurements=None
  C2 : powerlib/Elements/Series RLC Branch  LConnTagsString=__new0  RConnTagsString=__new0  BranchType=LC  Resistance=1  Inductance=200e-6  SetiL0=off  InitialCurrent=0  Capacitance=0.02027e-7  Setx0=off  InitialVoltage=0  Measurements=None
  Current Measurement1 : powerlib/Measurements/Current Measurement  PhasorSimulation=off  OutputType=Complex  PSBequivalent=0
  DC Voltage Source1 : powerlib/Electrical Sources/DC Voltage Source  Amplitude=190  Measurements=None
  DC Voltage Source2 : powerlib/Electrical Sources/DC Voltage Source  Amplitude=190  Measurements=None
  Display : Display
  Display1 : Display
  Mean : dspstat3/Mean  run=off  reset_popup=None  InputProcessing=Columns as channels (frame based)  directionMode=Each column  dimension=1  roiEnable=off  roiType=Rectangles  roiPortion=Entire ROI  roiOutput=Individual statistics for each ROI  roiFlag=off  outputDataTypeStr=Inherit: Same as accumulator  outputLastDataTypeStr=Inherit: Same as accumulator  outputMin=[]  outputMax=[]  roundingMode=Floor  overflowMode=off
  Mean1 : dspstat3/Mean  run=off  reset_popup=None  InputProcessing=Columns as channels (frame based)  directionMode=Each column  dimension=1  roiEnable=off  roiType=Rectangles  roiPortion=Entire ROI  roiOutput=Individual statistics for each ROI  roiFlag=off  outputDataTypeStr=Inherit: Same as accumulator  outputLastDataTypeStr=Inherit: Same as accumulator  outputMin=[]  outputMax=[]  roundingMode=Floor  overflowMode=off
  Mosfet : powerlib/Power Electronics/Mosfet  Ron=130e-3  Lon=0  Rd=0.25  Vfd=2.2  IC=0  Rs=1e5  Cs=inf  Measurements=off
  Mosfet1 : powerlib/Power Electronics/Mosfet  Ron=130e-3  Lon=0  Rd=0.25  Vfd=2.2  IC=0  Rs=1e5  Cs=inf  Measurements=off
  Rload : powerlib/Elements/Series RLC Branch  LConnTagsString=__new0  RConnTagsString=__new0  BranchType=R  Resistance=6  Inductance=1e-3  SetiL0=off  InitialCurrent=0  Capacitance=1e-6  Setx0=off  InitialVoltage=0  Measurements=None
  Scope : Scope  NumInputPorts=3
  Scope1 : Scope  NumInputPorts=2
  Subsystem : Subsystem
  Universal Bridge : powerlib/Power Electronics/Universal Bridge  Arms=2  SnubberResistance=1e5  SnubberCapacitance=inf  Device=Diodes  Ron=1e-3  Lon=0  ForwardVoltages="[  0  0  ]"  ForwardVoltage=0  GTOparameters=[ 10e-6 , 20e-6 ]  IGBTparameters=[ 1e-6 , 2e-6 ]  Measurements=None  Measurements_2=None  converterType=Rectifier
  Voltage Measurement : powerlib/Measurements/Voltage Measurement  PhasorSimulation=off  OutputType=Complex  PSBequivalent=0
  Voltage Measurement1 : powerlib/Measurements/Voltage Measurement  PhasorSimulation=off  OutputType=Complex  PSBequivalent=0
  Load AverageVoltage : Outport
  Load Average Current : Outport  Port=2
  wires:
  Mean/1 -> Load AverageVoltage/1, Display/1
  Subsystem/1("g1 ") -> [g1]
  Subsystem/2(g2) -> [g2]
  [g1] -> Mosfet/1, Scope1/1  "gate"
  [iload] -> Mean/1, Scope/3  "Iload"
  [loadV] -> Mean1/1, Scope/1  "Vload"
  [GaNV] -> Scope/2  "VGaN"
  Voltage Measurement/1 -> [loadV]
  [g2] -> Mosfet1/1
  Voltage Measurement1/1 -> [GaNV], Scope1/2  "voltage"
  Current Measurement1/1 -> [iload]
  Mean1/1 -> Load Average Current/1, Display1/1
  connections:
  C2/RConn1 -- Universal Bridge/LConn1
  Voltage Measurement/LConn2 -- Rload/RConn1 -- C1/RConn1 -- Universal Bridge/RConn2
  Universal Bridge/RConn1 -- C1/LConn1 -- Current Measurement1/LConn1
  Voltage Measurement1/LConn2 -- C2/LConn1 -- Mosfet1/LConn1 -- Mosfet/RConn1
  Voltage Measurement1/LConn1 -- DC Voltage Source1/RConn1 -- Mosfet/LConn1
  DC Voltage Source1/LConn1 -- Universal Bridge/LConn2 -- DC Voltage Source2/RConn1
  Voltage Measurement/LConn1 -- Current Measurement1/RConn1 -- Rload/LConn1
  DC Voltage Source2/LConn1 -- Mosfet1/RConn1

== system ResonantConverter_GaN/250 khz Switch1 ==
  note: Without a traansformer
  C1 : powerlib/Elements/Series RLC Branch  LConnTagsString=__new0  RConnTagsString=__new0  BranchType=C  Resistance=1  Inductance=1e-3  SetiL0=off  InitialCurrent=0  Capacitance=47e-6  Setx0=off  InitialVoltage=0  Measurements=None
  C2 : powerlib/Elements/Series RLC Branch  LConnTagsString=__new0  RConnTagsString=__new0  BranchType=LC  Resistance=1  Inductance=100e-6  SetiL0=off  InitialCurrent=0  Capacitance=0.02027e-7*2  Setx0=off  InitialVoltage=0  Measurements=None
  Current Measurement1 : powerlib/Measurements/Current Measurement  PhasorSimulation=off  OutputType=Complex  PSBequivalent=0
  DC Voltage Source1 : powerlib/Electrical Sources/DC Voltage Source  Amplitude=190  Measurements=None
  DC Voltage Source2 : powerlib/Electrical Sources/DC Voltage Source  Amplitude=190  Measurements=None
  Display : Display
  Display1 : Display
  Mean : dspstat3/Mean  run=off  reset_popup=None  InputProcessing=Columns as channels (frame based)  directionMode=Each column  dimension=1  roiEnable=off  roiType=Rectangles  roiPortion=Entire ROI  roiOutput=Individual statistics for each ROI  roiFlag=off  outputDataTypeStr=Inherit: Same as accumulator  outputLastDataTypeStr=Inherit: Same as accumulator  outputMin=[]  outputMax=[]  roundingMode=Floor  overflowMode=off
  Mean1 : dspstat3/Mean  run=off  reset_popup=None  InputProcessing=Columns as channels (frame based)  directionMode=Each column  dimension=1  roiEnable=off  roiType=Rectangles  roiPortion=Entire ROI  roiOutput=Individual statistics for each ROI  roiFlag=off  outputDataTypeStr=Inherit: Same as accumulator  outputLastDataTypeStr=Inherit: Same as accumulator  outputMin=[]  outputMax=[]  roundingMode=Floor  overflowMode=off
  Mosfet : powerlib/Power Electronics/Mosfet  Ron=130e-3  Lon=0  Rd=0.25  Vfd=2.2  IC=0  Rs=1e5  Cs=inf  Measurements=off
  Mosfet1 : powerlib/Power Electronics/Mosfet  Ron=130e-3  Lon=0  Rd=0.25  Vfd=2.2  IC=0  Rs=1e5  Cs=inf  Measurements=off
  Rload : powerlib/Elements/Series RLC Branch  LConnTagsString=__new0  RConnTagsString=__new0  BranchType=R  Resistance=6  Inductance=1e-3  SetiL0=off  InitialCurrent=0  Capacitance=1e-6  Setx0=off  InitialVoltage=0  Measurements=None
  Scope : Scope  NumInputPorts=3
  Scope1 : Scope  NumInputPorts=2
  Subsystem : Subsystem
  Universal Bridge : powerlib/Power Electronics/Universal Bridge  Arms=2  SnubberResistance=1e5  SnubberCapacitance=inf  Device=Diodes  Ron=1e-3  Lon=0  ForwardVoltages="[  0  0  ]"  ForwardVoltage=0  GTOparameters=[ 10e-6 , 20e-6 ]  IGBTparameters=[ 1e-6 , 2e-6 ]  Measurements=None  Measurements_2=None  converterType=Rectifier
  Voltage Measurement : powerlib/Measurements/Voltage Measurement  PhasorSimulation=off  OutputType=Complex  PSBequivalent=0
  Voltage Measurement1 : powerlib/Measurements/Voltage Measurement  PhasorSimulation=off  OutputType=Complex  PSBequivalent=0
  Load AverageVoltage : Outport
  Load Average Current : Outport  Port=2
  wires:
  Mean1/1 -> Display1/1, Load Average Current/1
  Current Measurement1/1 -> [iload]
  Voltage Measurement1/1 -> Scope1/2, [GaNV]  "voltage"
  [g2] -> Mosfet1/1
  Voltage Measurement/1 -> [loadV]
  [GaNV] -> Scope/2  "VGaN"
  [loadV] -> Scope/1, Mean1/1  "Vload"
  [iload] -> Scope/3, Mean/1  "Iload"
  [g1] -> Scope1/1, Mosfet/1  "gate"
  Subsystem/2(g2) -> [g2]
  Subsystem/1("g1 ") -> [g1]
  Mean/1 -> Display/1, Load AverageVoltage/1
  connections:
  DC Voltage Source2/LConn1 -- Mosfet1/RConn1
  Current Measurement1/RConn1 -- Voltage Measurement/LConn1 -- Rload/LConn1
  Universal Bridge/LConn2 -- DC Voltage Source1/LConn1 -- DC Voltage Source2/RConn1
  DC Voltage Source1/RConn1 -- Voltage Measurement1/LConn1 -- Mosfet/LConn1
  C2/LConn1 -- Mosfet1/LConn1 -- Voltage Measurement1/LConn2 -- Mosfet/RConn1
  C1/LConn1 -- Universal Bridge/RConn1 -- Current Measurement1/LConn1
  C1/RConn1 -- Universal Bridge/RConn2 -- Voltage Measurement/LConn2 -- Rload/RConn1
  C2/RConn1 -- Universal Bridge/LConn1

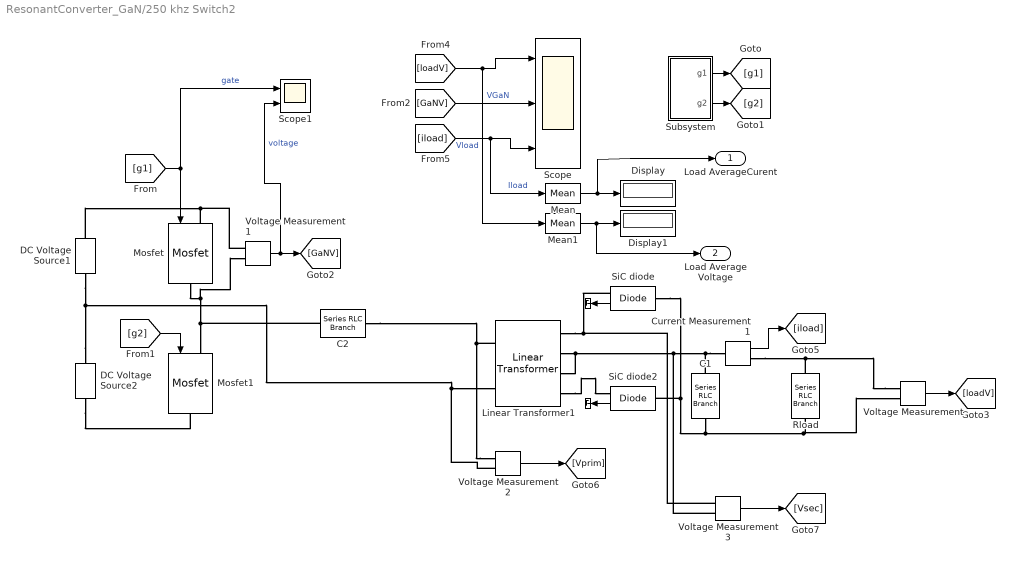
== system ResonantConverter_GaN/250 khz Switch2 ==
  "  " : Terminator
  "   " : Terminator
  C1 : powerlib/Elements/Series RLC Branch  LConnTagsString=__new0  RConnTagsString=__new0  BranchType=C  Resistance=1  Inductance=1e-3  SetiL0=off  InitialCurrent=0  Capacitance=1e-6  Setx0=off  InitialVoltage=0  Measurements=None
  C2 : powerlib/Elements/Series RLC Branch  LConnTagsString=__new0  RConnTagsString=__new0  BranchType=LC  Resistance=1  Inductance=100e-6  SetiL0=off  InitialCurrent=0  Capacitance=0.02027e-7*2  Setx0=off  InitialVoltage=0  Measurements=None
  Current Measurement1 : powerlib/Measurements/Current Measurement  PhasorSimulation=off  OutputType=Complex  PSBequivalent=0
  DC Voltage Source1 : powerlib/Electrical Sources/DC Voltage Source  Amplitude=190  Measurements=None
  DC Voltage Source2 : powerlib/Electrical Sources/DC Voltage Source  Amplitude=190  Measurements=None
  Display : Display
  Display1 : Display
  Linear Transformer1 : powerlib/Elements/Linear Transformer  UNITS=SI  NominalPower=[ 400 250e3 ]  winding1=[190 0.6e-3 25e-09]  winding2=[190 0.6e-3 25e-09]  ThreeWindings=on  winding3=[190 0.6e-3 25e-09]  RmLm=[4500 700e-06]  Measurements=None  DataType=on
  Mean : dspstat3/Mean  run=off  reset_popup=None  InputProcessing=Columns as channels (frame based)  directionMode=Each column  dimension=1  roiEnable=off  roiType=Rectangles  roiPortion=Entire ROI  roiOutput=Individual statistics for each ROI  roiFlag=off  outputDataTypeStr=Inherit: Same as accumulator  outputLastDataTypeStr=Inherit: Same as accumulator  outputMin=[]  outputMax=[]  roundingMode=Floor  overflowMode=off
  Mean1 : dspstat3/Mean  run=off  reset_popup=None  InputProcessing=Columns as channels (frame based)  directionMode=Each column  dimension=1  roiEnable=off  roiType=Rectangles  roiPortion=Entire ROI  roiOutput=Individual statistics for each ROI  roiFlag=off  outputDataTypeStr=Inherit: Same as accumulator  outputLastDataTypeStr=Inherit: Same as accumulator  outputMin=[]  outputMax=[]  roundingMode=Floor  overflowMode=off
  Mosfet : powerlib/Power Electronics/Mosfet  Ron=130e-3  Lon=0  Rd=0.25  Vfd=2.2  IC=0  Rs=1e5  Cs=inf  Measurements=off
  Mosfet1 : powerlib/Power Electronics/Mosfet  Ron=130e-3  Lon=0  Rd=0.25  Vfd=2.2  IC=0  Rs=1e5  Cs=inf  Measurements=off
  Rload : powerlib/Elements/Series RLC Branch  LConnTagsString=__new0  RConnTagsString=__new0  BranchType=R  Resistance=6  Inductance=1e-3  SetiL0=off  InitialCurrent=0  Capacitance=1e-6  Setx0=off  InitialVoltage=0  Measurements=None
  Scope : Scope  NumInputPorts=3
  Scope1 : Scope  NumInputPorts=2
  SiC diode : powerlib/Power Electronics/Diode  Ron=0.001  Lon=0  Vf=0.8  IC=0  UseSnubber=off  Rs=500  Cs=250e-9  Measurements=on
  SiC diode2 : powerlib/Power Electronics/Diode  Ron=0.001  Lon=0  Vf=0.8  IC=0  UseSnubber=off  Rs=500  Cs=250e-9  Measurements=on
  Subsystem : Subsystem
  Voltage Measurement{,1..3} (4 alike) : powerlib/Measurements/Voltage Measurement  PhasorSimulation=off  OutputType=Complex  PSBequivalent=0
  Load AverageCurent : Outport
  Load Average Voltage : Outport  Port=2
  wires:
  Mean/1 -> Load AverageCurent/1, Display/1
  Subsystem/1("g1 ") -> [g1]
  Subsystem/2(g2) -> [g2]
  [g1] -> Mosfet/1, Scope1/1  "gate"
  [iload] -> Mean/1, Scope/3  "Iload"
  [loadV] -> Mean1/1, Scope/1  "Vload"
  [GaNV] -> Scope/2  "VGaN"
  [g2] -> Mosfet1/1
  Voltage Measurement1/1 -> [GaNV], Scope1/2  "voltage"
  Mean1/1 -> Load Average Voltage/1, Display1/1
  Voltage Measurement/1 -> [loadV]
  Current Measurement1/1 -> [iload]
  SiC diode/1 -> "  "/1
  SiC diode2/1 -> "   "/1
  Voltage Measurement2/1 -> [Vprim]
  Voltage Measurement3/1 -> [Vsec]
  connections:
  Mosfet/RConn1 -- Voltage Measurement1/LConn2 -- Mosfet1/LConn1 -- C2/LConn1
  Mosfet/LConn1 -- Voltage Measurement1/LConn1 -- DC Voltage Source1/RConn1
  DC Voltage Source2/LConn1 -- Mosfet1/RConn1
  Voltage Measurement2/LConn1 -- C2/RConn1 -- Linear Transformer1/LConn1
  SiC diode/RConn1 -- Linear Transformer1/RConn1 -- Voltage Measurement3/LConn1
  Rload/RConn1 -- SiC diode/LConn1 -- SiC diode2/LConn1 -- C1/RConn1 -- Voltage Measurement/LConn2
  Voltage Measurement/LConn1 -- Current Measurement1/RConn1 -- Rload/LConn1
  Current Measurement1/LConn1 -- C1/LConn1 -- Voltage Measurement3/LConn2 -- Linear Transformer1/RConn3 -- Linear Transformer1/RConn2
  Linear Transformer1/RConn4 -- SiC diode2/RConn1
  DC Voltage Source2/RConn1 -- Voltage Measurement2/LConn2 -- Linear Transformer1/LConn2 -- DC Voltage Source1/LConn1
